simulink model "asm"  (R2018a)
settings: Solver=FixedStepAuto  StartTime=0.0  StopTime=3  FixedStep=0.01  RelTol=1e-3
libraries: aerolibactuator x2
settings Model: Creator=Ducted Fan  LastModifiedBy=Ducted Fan

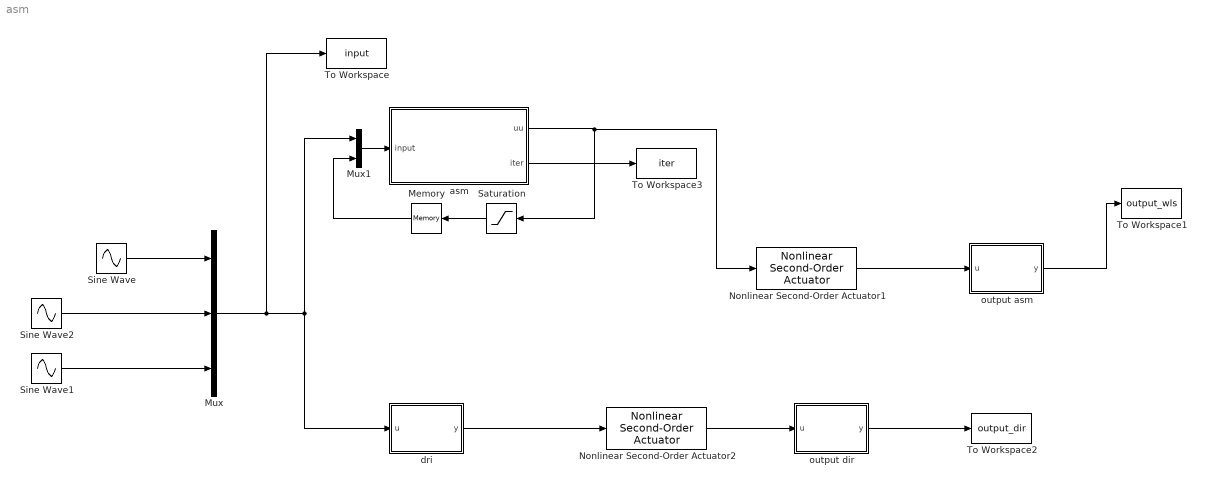
== system asm ==
  Memory : Memory  InitialCondition=[0;0;0;0]  InheritSampleTime=on  LinearizeAsDelay=on
  Mux : Mux  Inputs=3
  Mux1 : Mux  Inputs=2
  Nonlinear Second-Order Actuator1 : aerolibactuator/Nonlinear Second-Order Actuator  wn_fin=100  z_fin=1  fin_max=60*pi/180  fin_min=-60*pi/180  fin_maxrate=380*pi/180  fin_act_0=0  fin_act_vel=0
      settings: SourceProductName=Aerospace Blockset  SourceProductBaseCode=AE
  Nonlinear Second-Order Actuator2 : aerolibactuator/Nonlinear Second-Order Actuator  wn_fin=100  z_fin=1  fin_max=60*pi/180  fin_min=-60*pi/180  fin_maxrate=380*pi/180  fin_act_0=0  fin_act_vel=0
      settings: SourceProductName=Aerospace Blockset  SourceProductBaseCode=AE
  Saturation : Saturate  UpperLimit=[0.3491;0.3491;0.3491;0.3491]  LowerLimit=-[0.3491;0.3491;0.3491;0.3491]
  Sine Wave : Sin  Amplitude=0.33  Frequency=2*pi/2  SampleTime=0
  Sine Wave1 : Sin  Amplitude=0.17  Frequency=2*pi/2  SampleTime=0
  Sine Wave2 : Sin  Amplitude=0.34  Frequency=2*pi/2  Phase=pi/2  SampleTime=0
  To Workspace : ToWorkspace  VariableName=input  SaveFormat=Timeseries  SampleTime=-1
  To Workspace1 : ToWorkspace  VariableName=output_wls  SaveFormat=Timeseries  SampleTime=-1
  To Workspace2 : ToWorkspace  VariableName=output_dir  SaveFormat=Timeseries  SampleTime=-1
  To Workspace3 : ToWorkspace  VariableName=iter  SaveFormat=Timeseries  SampleTime=-1
  asm : MATLAB Function  TreatAsAtomicUnit=on
  dri : MATLAB Function  TreatAsAtomicUnit=on
  output asm : MATLAB Function  TreatAsAtomicUnit=on
  output dir : MATLAB Function  TreatAsAtomicUnit=on
  wires:
  Sine Wave2/1 -> Mux/2
  Sine Wave1/1 -> Mux/3
  Sine Wave/1 -> Mux/1
  Mux1/1 -> asm/1(input)
  output asm/1(y) -> To Workspace1/1
  Mux/1 -> To Workspace/1, dri/1(u), Mux1/1
  Memory/1 -> Mux1/2
  Saturation/1 -> Memory/1
  output dir/1(y) -> To Workspace2/1
  asm/1(uu) -> Nonlinear Second-Order Actuator1/1, Saturation/1
  dri/1(y) -> Nonlinear Second-Order Actuator2/1
  Nonlinear Second-Order Actuator1/1 -> output asm/1(u)
  Nonlinear Second-Order Actuator2/1 -> output dir/1(u)
  asm/2(iter) -> To Workspace3/1

== matlab function asm/output asm ==
  data: u input; y output
function y = fcn(u)
u(1)=Constrain(u(1),-0.3491,0.3491);
u(2)=Constrain(u(2),-0.3491,0.3491);
u(3)=Constrain(u(3),-0.3491,0.3491);
u(4)=Constrain(u(4),-0.3491,0.3491);
B=[-0.5   0       0.5   0;
    0  -0.5    0       0.5;
    0.25   0.25   0.25   0.25];
y = B*u;

== matlab function asm/dri ==
  data: u input; y output
function y = fcn(u)
e = [u(1);u(2);u(3)];
% M=crossover_point([0;0;0],e);
% if (norm(e)>norm(M))
%     U=M;
% else
%     U=e;
% end 
B=[-0.5   0       0.5   0;
    0  -0.5    0       0.5;
    0.25   0.25   0.25   0.25];
% u(1)=Constrain(u(1),umin(1),umax(1));
% u(2)=Constrain(u(2),umin(2),umax(2));
% u(3)=Constrain(u(3),umin(3),umax(3));
% u(4)=Constrain(u(4),umin(4),umax(4));
y=pinv(B)*e;

== matlab function asm/output dir ==
  data: u input; y output
function y = fcn(u)
u(1)=Constrain(u(1),-0.3491,0.3491);
u(2)=Constrain(u(2),-0.3491,0.3491);
u(3)=Constrain(u(3),-0.3491,0.3491);
u(4)=Constrain(u(4),-0.3491,0.3491);
B=[-0.5   0       0.5   0;
    0  -0.5    0       0.5;
    0.25   0.25   0.25   0.25];
y = B*u;

== matlab function asm/asm ==
  data: input input; uu output; iter output
function [uu ,iter]= wls_alloc(input)
v=[input(1);input(2);input(3)];
% M=crossover_point([0;0;0],e);
% if (norm(e)>norm(M))
%     v=M;
% else
%     v=e;
% end 
u_last=zeros(4,1);
u_last=[input(4);input(5);input(6);input(7)];
uu=u_last;
% WLS_ALLOC - Control allocation using weighted least squares.
%
%  [u,W,iter] = wls_alloc(B,v,umin,umax,[Wv,Wu,ud,gamma,u0,W0,imax])
%
% Solves the weighted, bounded least-squares problem
%
%   min ||Wu(u-ud)||^2 + gamma ||Wv(Bu-v)||^2
%
%   subj. to  umin <= u <= umax
%
% using an active set method.
%
%  Inputs:
%  -------
% v     commanded virtual control (k x 1)
% u0    initial point (m x 1)
% W0    initial working set (m x 1) [empty]
% imax  max no. of iterations [100]
%
%  Outputs:
%  -------
% u     optimal control
% W     optimal active set
% iter  no. of iterations (= no. of changes in the working set + 1)
%
%                            0 if u_i not saturated
% Working set syntax: W_i = -1 if u_i = umin_i
%                           +1 if u_i = umax_i
%
% B         control effectiveness matrix (k x m).
% umin      lower position limits (m x 1).
% umax      upper position limits (m x 1).
% Wv        virtual control weighting matrix (k x k) [I].
% Wu        control weighting matrix (m x m) [I].
% gam       gamma weight (scalar) [1e6].
% ud        desired control (m x 1) [0].
% imax      maximum iterations.
% 
% See also: WLSC_ALLOC, IP_ALLOC, FXP_ALLOC, QP_SIM.

% param of ducted fan
% ======================multi ducted fan param=========================
% kc=3.157;
% l_1=0.17078793-0.09;% roll,pitch
% l_2=0.175;% T
% l_3=0.06647954;% yaw1 yaw3
% l_4=0.06647954+0.175;% yaw4
% l_5=0.175-0.06647954;% yaw2
% I_x=0.054593;
% I_y=0.017045;
% I_z=0.049226;
% I=[I_x 0 0;0 I_y 0;0 0 I_z];
% =========================10 sureface=================================
% K=[-kc*l_1/5 0 kc*l_1/5 0 -kc*l_1/5 0 kc*l_1/5 0 2*l_2/5;
%     0 -kc*l_1/4 0 kc*l_1/4 0 -kc*l_1/4 0 kc*l_1/4 0;
%     kc*l_3/8 -kc*l_5/8 kc*l_3/8 kc*l_4/8 kc*l_3/8 kc*l_4/8 kc*l_3/8 -kc*l_5/8 0];
% B=I\K;
% umin=[[1;1;1;1;1;1;1;1]*-20*pi/180;-0.3*9.788];umax=[[1;1;1;1;1;1;1;1]*20*pi/180;0.3*9.788];
% Wu=eye(9);
% ud=zeros(9,1);
% % Number of variables.
% m = 9;
%===================================================
% =========================8 sureface=================================
% K=[-kc*l_1/4 0 kc*l_1/4 0 -kc*l_1/4 0 kc*l_1/4 0;
%     0 -kc*l_1/4 0 kc*l_1/4 0 -kc*l_1/4 0 kc*l_1/4;
%     kc*l_3/8 -kc*l_5/8 kc*l_3/8 kc*l_4/8 kc*l_3/8 kc*l_4/8 kc*l_3/8 -kc*l_5/8 ];
% B=I\K;
% umin=[1;1;1;1;1;1;1;1]*-20*pi/180;umax=[1;1;1;1;1;1;1;1]*20*pi/180;
% Wu=eye(8);
% ud=zeros(8,1);
% % Number of variables.
% m = 8;
%========================================
% K=[-kc*l_1/4    -kc*l_1/4   0           kc*l_1/4    kc*l_1/4    0;
%     0           0           -kc*l_1/2   0           0           kc*l_1/2;
%     kc*l_3/6    kc*l_3/6    kc*l_4/6    kc*l_3/6    kc*l_3/8    kc*l_4/6 ];
% B=I\K;
% umin=[1;1;1;1;1;1]*-20*pi/180;umax=[1;1;1;1;1;1]*20*pi/180;
% Wu=eye(6);
% ud=zeros(6,1);
% % Number of variables.
% m = 6;
%============================
B=[-0.5   0       0.5   0;
    0  -0.5    0       0.5;
    0.25   0.25   0.25   0.25];


umin=max([1;1;1;1]*(-20)*pi/180,-5*pi/180+u_last);
umax=min([1;1;1;1]*20*pi/180,5*pi/180+u_last);
%========有效集的重新初始化============
W=zeros(4,1);
infeasible1 = (uu < umin);
W(infeasible1)=-1;
infeasible2 = (uu > umax);
W(infeasible2)= 1;
%=======================================
% umin=[1;1;1;1]*(-20)*pi/180;
% umax=[1;1;1;1]*20*pi/180;
ud=[0;0;0;0];
% Number of variables.
m = 4;
%================================
% 加权系数
gam=1e6;
% 加权矩阵
Wv=eye(3);
Wu=eye(4);
% 迭代次数上限
imax=100;
% Set default values of optional arguments.
gam_sq = sqrt(gam);
A = [gam_sq*Wv*B ; Wu];
b = [gam_sq*Wv*v ; Wu*ud];

% Initial residual.
d = b - A*uu;
% Determine indeces of free variables.
i_free = W==0;

% Iterate until optimum is found or maximum number of iterations
% is reached.

for iter = 1:imax
    % ----------------------------------------
    %  Compute optimal perturbation vector p.
    % ----------------------------------------
    % Eliminate saturated variables.
    A_free = A(:,i_free);
    % Solve the reduced optimization problem for free variables.
    p_free = A_free\d;
    % Zero all perturbations corresponding to active constraints.
    p = zeros(m,1);
    % Insert perturbations from p_free into free the variables.
    p(i_free) = p_free;
    
    % ----------------------------
    %  Is the new point feasible?
    % ----------------------------
    
    u_opt = uu + p;
    infeasible = (u_opt < umin) | (u_opt > umax);
    
    if ~any(infeasible(i_free))
        
        % ----------------------------
        %  Yes, check for optimality.
        % ----------------------------
        
        % Update point and residual.
        uu = u_opt;
        d = d - A_free*p_free;
        if norm(p)<=eps
        % Compute Lagrangian multipliers.
        lambda = W.*(A'*d);
        % Are all lambda non-negative?
        if lambda >= -eps
            % / ------------------------ \
            % | Optimum found, bail out. |
            % \ ------------------------ /
            return;
        end
        
        % --------------------------------------------------
        %  Optimum not found, remove one active constraint.
        % --------------------------------------------------
        
        % Remove constraint with most negative lambda from the
        % working set.
        [~,i_neg] = min(lambda);
        W(i_neg) = 0;
        i_free(i_neg) = 1;
        end
    else
        
        % ---------------------------------------
        %  No, find primary bounding constraint.
        % ---------------------------------------
        
        % Compute distances to the different boundaries. Since alpha < 1 is
        % the maximum step length, initiate with ones.
        dist = ones(m,1);
        i_min = i_free & p<0;
        i_max = i_free & p>0;
        dist(i_min) = (umin(i_min) - uu(i_min)) ./ p(i_min);
        dist(i_max) = (umax(i_max) - uu(i_max)) ./ p(i_max);
        
        % Proportion of p to travel
        [alpha,i_alpha] = min(dist);
        % Update point and residual.
        uu = uu + alpha*p;
        % Update point and residual.
        d = d - A_free*alpha*p_free;
        
        % Add corresponding constraint to working set.
        W(i_alpha) = sign(p(i_alpha));
        i_free(i_alpha) = 0;
        
    end
    
end

end
